simulink subsystem "Find_Target_Pose"  (R2023b)
settings: Solver=VariableStepAuto  StartTime=0.0  StopTime=10.0  RelTol=1e-3
undefined symbols (not defined in the file): Spline_Capture_Radius, Spline_Max_Num_RefPoses
libraries: simulink x1
settings Model: Creator=FIRSTMentor  LastModifiedBy=ander

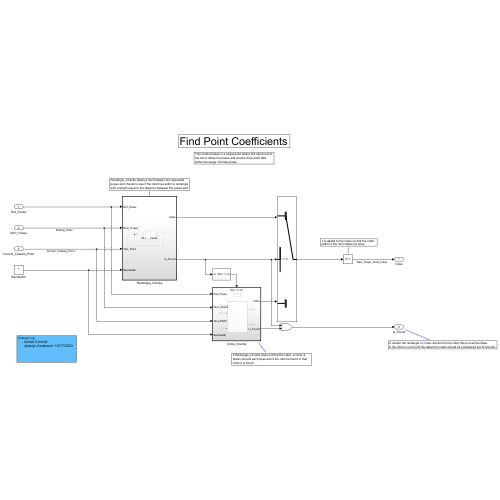
[thumbnail: Simulink's stored preview of the top-level diagram]
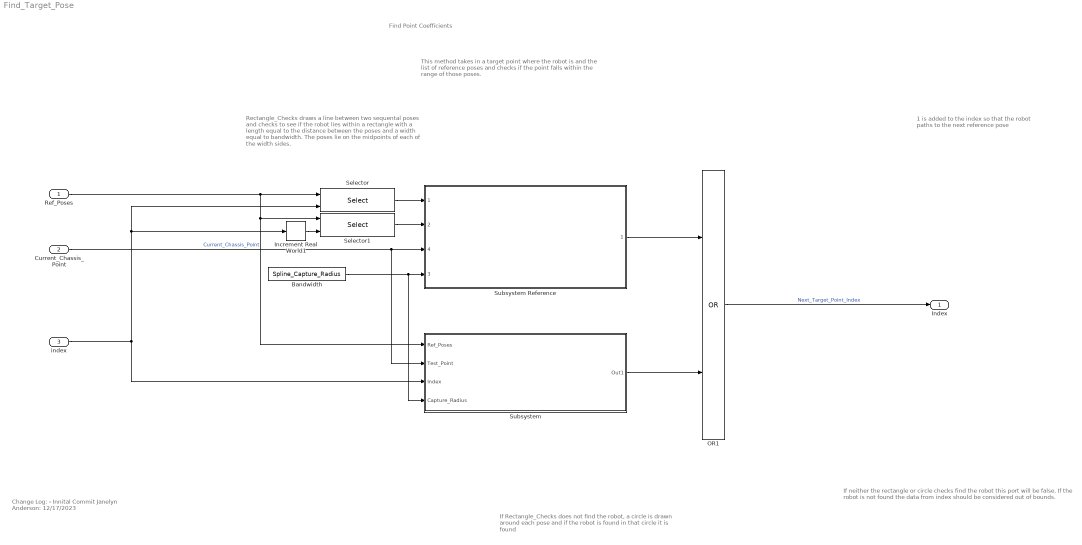
== system Find_Target_Pose ==
  note: 1 is added to the index so that the robot paths to the next reference pose
  note: If neither the rectangle or circle checks find the robot this port will be false.
      | If the robot is not found the data from index should be considered out of bounds.
  note: Change Log:
      | - Innital Commit
      | Janelyn Anderson: 12/17/2023
  note: Find Point Coefficients
  note: This method takes in a target point where the robot is and the list of reference poses and checks if the point falls within the range of those poses.
  note: Rectangle_Checks draws a line between two sequental poses and checks to see if the robot lies within a rectangle with a length equal to the distance between the poses and a width equal to bandwidth. The poses lie on the midpoints of each of the width sides.
  note: If Rectangle_Checks does not find the robot, a circle is drawn around each pose and if the robot is found in that circle it is found
  Ref_Poses : Inport  OutDataTypeStr=double  PortDimensions=[Spline_Max_Num_RefPoses 2]
  Current_Chassis_Point : Inport  Port=2  OutDataTypeStr=double  Unit=m  PortDimensions=[1 2]
  index : Inport  Port=3
  Bandwidth : Constant  Value=Spline_Capture_Radius
  Increment Real World1 : simulink/Additional Math & Discrete/Additional Math: Increment - Decrement/Increment Real World
  OR1 : Logic  Operator=OR  AllPortsSameDT=off  OutDataTypeStr=boolean
  Selector : Selector  NumberOfDimensions=2  InputPortWidth=3  IndexOptions=Index vector (port),Select all  Indices=[1 3],1  OutputSizes=1,1
  Selector1 : Selector  NumberOfDimensions=2  InputPortWidth=3  IndexOptions=Index vector (port),Select all  Indices=[1 3],1  OutputSizes=1,1
  Subsystem : Subsystem
  Subsystem Reference : Subsystem  ReferencedSubsystem=Bandwidth_Check_Between_Two_Points
      settings: PortSchema="{\"entries\":[{\"content\":{\"sides\":[{\"content\":{\"connectorIds\":[\"In1\",\"In2\",\"In4\",\"In3\"]},\"type\":\"ConnectorPlacement.EquallySpacedRectSide\",\"uuid\":\"ceb776b8-c050-4a98-93b2-29d0e514edc7\"},{\"content\":{\"connectorIds\":[\"Out1\"],\"side\":\"RIGHT\"},\"type\":\"ConnectorPlacement.EquallySpacedRectSide\",\"uuid\":\"6b0bd286-7e09-4672-ae75-d20305541db2\"},{\"content\":{\"side\":\"TOP\"},\"type\":\"ConnectorPlacement.EquallySpacedRectSide\",\"uuid\":\"2a1e7e93-e406-49f3-8e81-1c2419e85ee2\"}]},\"type\":\"ConnectorPlacement.EquallySpacedConnector\",\"uuid\":\"a612ddb7-ae02-43ab-a30c-20f014ad7d06\"}],\"packageUris\":[\"http://schema.mathworks.com/mf0/Connector/R2020b\"],\"version\":\"1.0\"}"
  Index : Outport
  wires:
  Current_Chassis_Point/1 -> Subsystem Reference/4, Subsystem/2(Test_Point)  "Current_Chassis_Point"
  Ref_Poses/1 -> Subsystem/1(Ref_Poses), Selector1/1, Selector/1
  OR1/1 -> Index/1  "Next_Target_Point_Index"
  Selector/1 -> Subsystem Reference/1
  Selector1/1 -> Subsystem Reference/2
  Increment Real World1/1 -> Selector1/2
  Bandwidth/1 -> Subsystem Reference/3, Subsystem/4(Capture_Radius)
  Subsystem Reference/1 -> OR1/1
  Subsystem/1(Out1) -> OR1/2
  index/1 -> Subsystem/3(Index), Selector/2, Increment Real World1/1

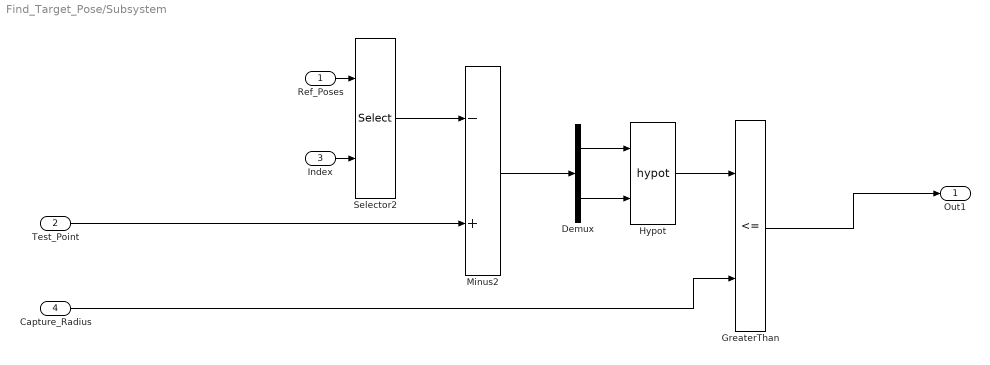
== system Find_Target_Pose/Subsystem ==
  Ref_Poses : Inport
  Test_Point : Inport  Port=2
  Index : Inport  Port=3
  Capture_Radius : Inport  Port=4
  Demux : Demux  Outputs=2
  GreaterThan : RelationalOperator  Operator=<=  OutDataTypeStr=boolean  RndMeth=Simplest  InputSameDT=off
  Hypot : Math  Operator=hypot
  Minus2 : Sum  Inputs=-+
  Selector2 : Selector  NumberOfDimensions=2  InputPortWidth=3  IndexOptions=Index vector (port),Select all  Indices=[1 3],1  OutputSizes=1,1
  Out1 : Outport
  wires:
  Index/1 -> Selector2/2
  GreaterThan/1 -> Out1/1
  Demux/2 -> Hypot/2
  Ref_Poses/1 -> Selector2/1
  Test_Point/1 -> Minus2/2
  Demux/1 -> Hypot/1
  Hypot/1 -> GreaterThan/1
  Selector2/1 -> Minus2/1
  Capture_Radius/1 -> GreaterThan/2
  Minus2/1 -> Demux/1
